simulink model "satelliteSim_KM"  (R2014a)
settings: Solver=ode45  StartTime=0.0  StopTime=10.0  RelTol=1e-3
values from neighbouring files (symbols this model uses):
  I = I+k    [E205_Lab4_satellite.m]    (also in satellitescript.m)
  J = 2    [E205_Lab4_satellite.m]    (also in satellitescript.m)
  Jhat = 1    [E205_Lab4_satellite.m]    (also in satellitescript.m)
  thetar = r    (= 1)    [E205_Lab4_satellite.m]    (also in satellitescript.m)
  thetardot = 0    [E205_Lab4_satellite.m]    (also in satellitescript.m)
  zeta = 1    [E205_Lab4_satellite.m]    (also in satellitescript.m)
undefined symbols (not defined in the file or in its folder): disturbance, mu_D, mu_P, wn
settings Model: Creator=Kristina  LastModifiedBy=Jessica
settings DebuggingCC: UnderspecifiedInitializationDetection=Classic

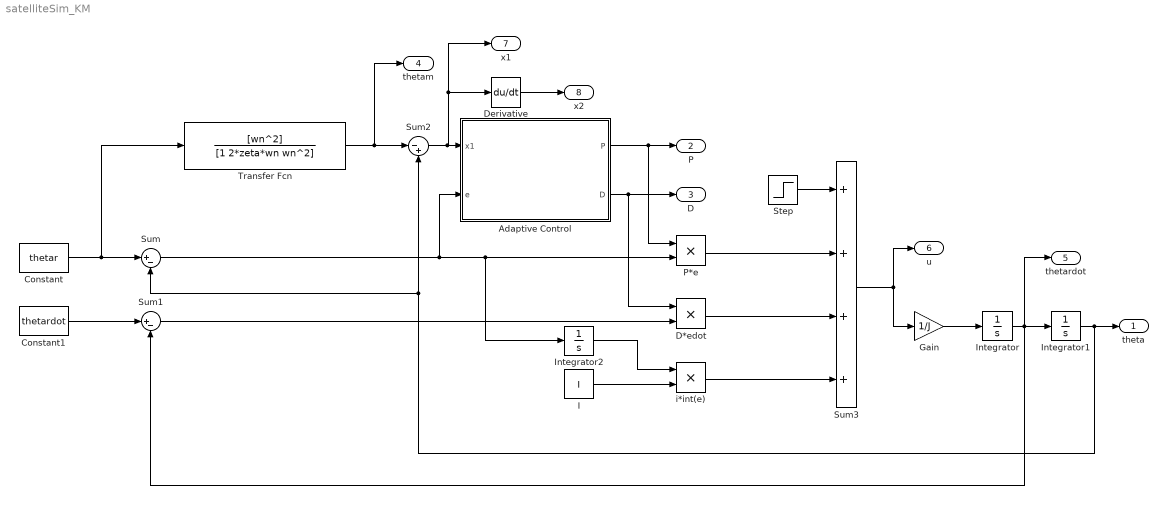
== system satelliteSim_KM ==
  Adaptive Control : Subsystem
  Constant : Constant  Value=thetar
  Constant1 : Constant  Value=thetardot
  D*edot : Product
  Derivative : Derivative
  Gain : Gain  Gain=1/J
  I : Constant  Value=I
  Integrator : Integrator
  Integrator1 : Integrator
  Integrator2 : Integrator
  P*e : Product
  Step : Step  Time=0  After=disturbance  SampleTime=0
  Sum : Sum  Inputs=|+-
  Sum1 : Sum  Inputs=|+-
  Sum2 : Sum  Inputs=|-+
  Sum3 : Sum  Inputs=++++
  Transfer Fcn : TransferFcn  Numerator=[wn^2]  Denominator=[1 2*zeta*wn wn^2]
  i*int(e) : Product
  theta : Outport
  P : Outport  Port=2
  D : Outport  Port=3
  thetam : Outport  Port=4
  thetardot : Outport  Port=5
  u : Outport  Port=6
  x1 : Outport  Port=7
  x2 : Outport  Port=8
  wires:
  Constant/1 -> Transfer Fcn/1, Sum/1
  Constant1/1 -> Sum1/1
  Sum/1 -> Adaptive Control/2(e), Integrator2/1, P*e/2
  Adaptive Control/1(P) -> P*e/1, P/1
  Adaptive Control/2(D) -> D*edot/1, D/1
  Sum1/1 -> D*edot/2
  D*edot/1 -> Sum3/3
  P*e/1 -> Sum3/2
  Sum3/1 -> Gain/1, u/1
  Gain/1 -> Integrator/1
  Integrator/1 -> thetardot/1, Integrator1/1, Sum1/2
  Integrator1/1 -> Sum/2, Sum2/2, theta/1
  Transfer Fcn/1 -> thetam/1, Sum2/1
  Sum2/1 -> Derivative/1, x1/1, Adaptive Control/1(x1)
  Derivative/1 -> x2/1
  I/1 -> i*int(e)/2
  Integrator2/1 -> i*int(e)/1
  i*int(e)/1 -> Sum3/4
  Step/1 -> Sum3/1

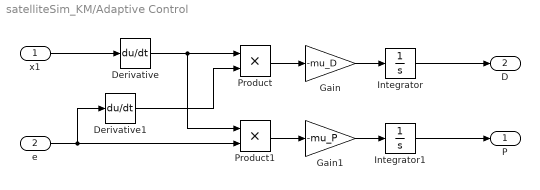
== system satelliteSim_KM/Adaptive Control ==
  x1 : Inport
  e : Inport  Port=2
  Derivative : Derivative
  Derivative1 : Derivative
  Gain : Gain  Gain=-mu_D
  Gain1 : Gain  Gain=-mu_P
  Integrator : Integrator  InitialCondition=Jhat*2*zeta*wn
  Integrator1 : Integrator  InitialCondition=Jhat*wn^2
  Product : Product
  Product1 : Product
  P : Outport
  D : Outport  Port=2
  wires:
  Integrator1/1 -> P/1
  x1/1 -> Derivative/1
  e/1 -> Product1/2, Derivative1/1
  Product/1 -> Gain/1
  Integrator/1 -> D/1
  Derivative/1 -> Product1/1, Product/1
  Gain1/1 -> Integrator1/1
  Derivative1/1 -> Product/2
  Product1/1 -> Gain1/1
  Gain/1 -> Integrator/1
